simulink model "V605_test_rig"  (R2025a)
settings: Solver=VariableStepAuto  StartTime=0.0  StopTime=100  RelTol=1e-3
libraries: simulink x1
settings Model: Creator=Ayush_S  LastModifiedBy=Ayush_S

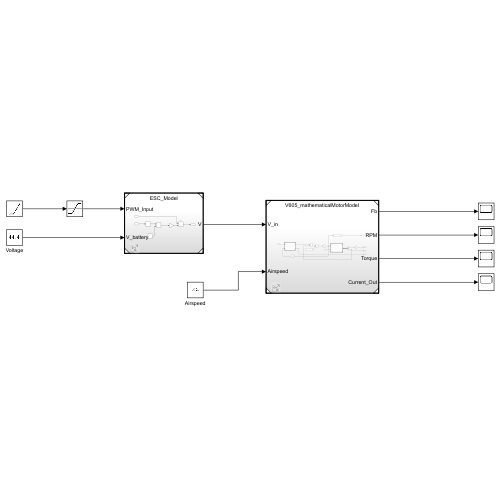
[thumbnail: Simulink's stored preview of the top-level diagram]
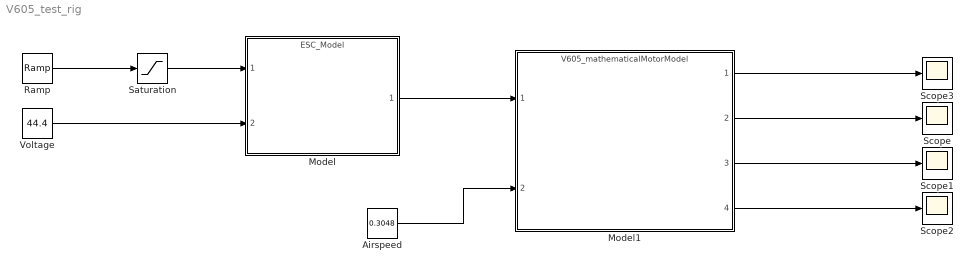
== system V605_test_rig ==
  Airspeed : Constant  Value=0.3048
  Model : ModelReference  ModelNameDialog=ESC_Model.slx  SimulationMode=Normal  ModelReferenceVersion=1.9
  Model1 : ModelReference  ModelNameDialog=V605_mathematicalMotorModel.slx  SimulationMode=Normal  ModelReferenceVersion=3.63
  Ramp : simulink/Sources/Ramp  slope=10  start=0  InitialOutput=1000
  Saturation : Saturate  UpperLimit=2000  LowerLimit=1000
  Scope{,1..3} (4 alike) : Scope
      Scope settings: ActiveDisplayYMinimum=-1775.3749615261449  ActiveDisplayYMaximum=12188.792094810477
      Scope1 settings: ActiveDisplayYMinimum=-3.0949507093541948  ActiveDisplayYMaximum=5.6138996622669213
      Scope2 settings: ActiveDisplayYMinimum=-18.911105064795066  ActiveDisplayYMaximum=202.71454930969355  DataLoggingVariableName=ScopeData2
      Scope3 settings: ActiveDisplayYMinimum=-108.8671405182115  ActiveDisplayYMaximum=156.46412243407946  DataLoggingVariableName=ScopeData3
  Voltage : Constant  Value=44.4
  wires:
  Model/1 -> Model1/1
  Voltage/1 -> Model/2
  Airspeed/1 -> Model1/2
  Model1/2 -> Scope/1
  Model1/1 -> Scope3/1
  Model1/3 -> Scope1/1
  Model1/4 -> Scope2/1
  Ramp/1 -> Saturation/1
  Saturation/1 -> Model/1
